simulink model "ThreePhaseInverter"  (R2020a)
settings: Solver=VariableStepAuto  StartTime=0.0  StopTime=0.1  RelTol=1e-3
libraries: powerlib x15, powerlib_meascontrol x6, simulink x4
settings Model: Creator=anif4  LastModifiedBy=anif4

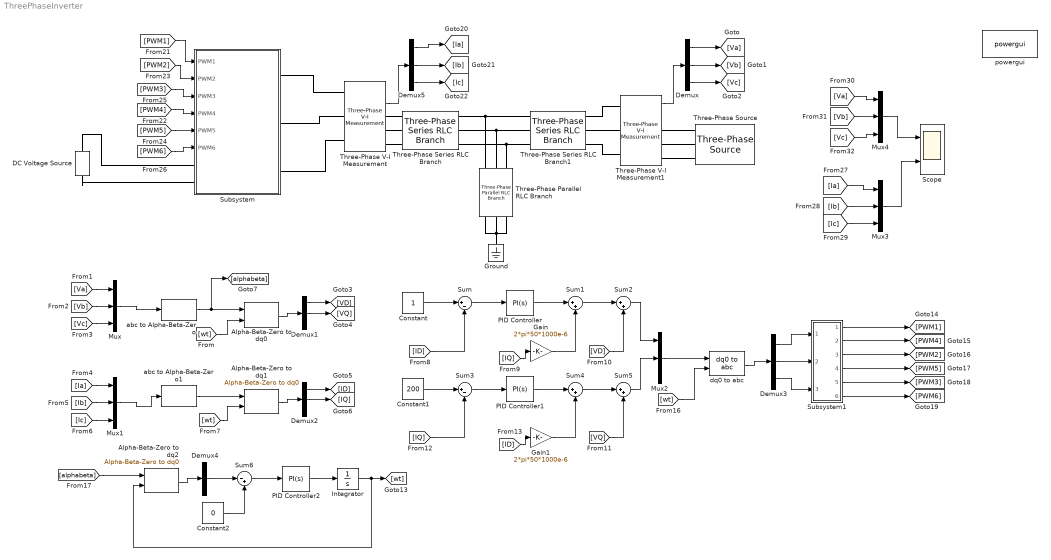
== system ThreePhaseInverter ==
  Alpha-Beta-Zero to dq0 : powerlib_meascontrol/Transformations/Alpha-Beta-Zero to dq0  Alignment=90 degrees behind phase A axis
  Alpha-Beta-Zero to dq1 : powerlib_meascontrol/Transformations/Alpha-Beta-Zero to dq0  Alignment=90 degrees behind phase A axis
  Alpha-Beta-Zero to dq2 : powerlib_meascontrol/Transformations/Alpha-Beta-Zero to dq0  Alignment=90 degrees behind phase A axis
  Constant : Constant
  Constant1 : Constant  Value=200
  Constant2 : Constant  Value=0
  DC Voltage Source : powerlib/Electrical Sources/DC Voltage Source  Amplitude=800  Measurements=None
  Demux{,1..5} (6 alike) : Demux  Outputs=3
  Gain : Gain  Gain=2*pi*50*1000e-6
  Gain1 : Gain  Gain=2*pi*50*1000e-6
  Ground : powerlib/Elements/Ground  LConnTagsString=a
  Integrator : Integrator
  Mux{,1..4} (5 alike) : Mux  Inputs=3
  PID Controller : simulink/Continuous/PID Controller  Controller=PI  Form=Parallel  TimeDomain=Continuous-time  UseExternalTs=off  SampleTime=-1  IntegratorMethod=Forward Euler  FilterMethod=Forward Euler  ControllerParametersSource=internal  P=5  I=5000  D=0  UseFilter=on  N=100  TunerSelectOption=Transfer Function Based (PID Tuner App)  InitialConditionSource=internal  InitialConditionForIntegrator=0  InitialConditionForFilter=0  DifferentiatorICPrevScaledInput=0  ExternalReset=none  TrackingMode=off  Kt=1  LimitOutput=off  UpperSaturationLimit=inf  LowerSaturationLimit=-inf  LinearizeAsGain=on  AntiWindupMode=none  Kb=1  POutMin=[]  POutMax=[]  IOutMin=[]  IOutMax=[]  DOutMin=[]  DOutMax=[]  NOutMin=[]  NOutMax=[]  SumOutMin=[]  SumOutMax=[]  SaturationOutMin=[]  SaturationOutMax=[]  PParamMin=[]  PParamMax=[]  IParamMin=[]  IParamMax=[]  DParamMin=[]  DParamMax=[]  NParamMin=[]  NParamMax=[]  KbParamMin=[]  KbParamMax=[]  KtParamMin=[]  KtParamMax=[]  KbOutMin=[]  KbOutMax=[]  KtOutMin=[]  KtOutMax=[]  IntegratorOutMin=[]  IntegratorOutMax=[]  FilterOutMin=[]  FilterOutMax=[]  SumI1OutMin=[]  SumI1OutMax=[]  SumI2OutMin=[]  SumI2OutMax=[]  SumI3OutMin=[]  SumI3OutMax=[]  SumI4OutMin=[]  SumI4OutMax=[]  SumDOutMin=[]  SumDOutMax=[]  DifferentiatorOutMin=[]  DifferentiatorOutMax=[]  FilterDiffOutCoefMin=[]  FilterDiffOutCoefMax=[]  ReciprocalOutMin=[]  ReciprocalOutMax=[]  SumDenOutMin=[]  SumDenOutMax=[]  SumNumOutMin=[]  SumNumOutMax=[]  DivideOutMin=[]  DivideOutMax=[]  UdiffTsProdOutMin=[]  UdiffTsProdOutMax=[]  NTsProdOutMin=[]  NTsProdOutMax=[]  UintegralTsProdOutMin=[]  UintegralTsProdOutMax=[]  UngainTsProdOutMin=[]  UngainTsProdOutMax=[]  IntegratorContinuousStateAttributes=''  IntegratorStateMustResolveToSignalObject=off  IntegratorRTWStateStorageClass=Auto  FilterContinuousStateAttributes=''  FilterStateMustResolveToSignalObject=off  FilterRTWStateStorageClass=Auto  ParallelPVariant=InternalParameters  IdealPVariant=Disabled  IVariant=InternalParameters  DVariant=Disabled  IntegratorVariant=Continuous  SatVariant=Disabled  AWVariant=Passthrough  PCopyVariant=Disabled  TRVariant=Disabled  FdbkBlocksVariant=Forward  IdealPFdbkVariant=Disabled  SatFdbkVariant=Disabled  DerivativeFilterVariant=Disabled  NVariant=Disabled  NCopyVariant=Disabled_SignalSpec  FilterICVariant=Disabled  IntegratorICVariant=InternalICs  ExternalResetVariant=Disabled  TRSumVariant=Passthrough  SumFdbkVariant=Disabled  SumVariant=Sum_PI  TsampFilterVariant=InternalTs  TsampNgainVariant=Passthrough  TsampIntegralVariant=Passthrough
  PID Controller1 : simulink/Continuous/PID Controller  Controller=PI  Form=Parallel  TimeDomain=Continuous-time  UseExternalTs=off  SampleTime=-1  IntegratorMethod=Forward Euler  FilterMethod=Forward Euler  ControllerParametersSource=internal  P=5  I=5000  D=0  UseFilter=on  N=100  TunerSelectOption=Transfer Function Based (PID Tuner App)  InitialConditionSource=internal  InitialConditionForIntegrator=0  InitialConditionForFilter=0  DifferentiatorICPrevScaledInput=0  ExternalReset=none  TrackingMode=off  Kt=1  LimitOutput=off  UpperSaturationLimit=inf  LowerSaturationLimit=-inf  LinearizeAsGain=on  AntiWindupMode=none  Kb=1  POutMin=[]  POutMax=[]  IOutMin=[]  IOutMax=[]  DOutMin=[]  DOutMax=[]  NOutMin=[]  NOutMax=[]  SumOutMin=[]  SumOutMax=[]  SaturationOutMin=[]  SaturationOutMax=[]  PParamMin=[]  PParamMax=[]  IParamMin=[]  IParamMax=[]  DParamMin=[]  DParamMax=[]  NParamMin=[]  NParamMax=[]  KbParamMin=[]  KbParamMax=[]  KtParamMin=[]  KtParamMax=[]  KbOutMin=[]  KbOutMax=[]  KtOutMin=[]  KtOutMax=[]  IntegratorOutMin=[]  IntegratorOutMax=[]  FilterOutMin=[]  FilterOutMax=[]  SumI1OutMin=[]  SumI1OutMax=[]  SumI2OutMin=[]  SumI2OutMax=[]  SumI3OutMin=[]  SumI3OutMax=[]  SumI4OutMin=[]  SumI4OutMax=[]  SumDOutMin=[]  SumDOutMax=[]  DifferentiatorOutMin=[]  DifferentiatorOutMax=[]  FilterDiffOutCoefMin=[]  FilterDiffOutCoefMax=[]  ReciprocalOutMin=[]  ReciprocalOutMax=[]  SumDenOutMin=[]  SumDenOutMax=[]  SumNumOutMin=[]  SumNumOutMax=[]  DivideOutMin=[]  DivideOutMax=[]  UdiffTsProdOutMin=[]  UdiffTsProdOutMax=[]  NTsProdOutMin=[]  NTsProdOutMax=[]  UintegralTsProdOutMin=[]  UintegralTsProdOutMax=[]  UngainTsProdOutMin=[]  UngainTsProdOutMax=[]  IntegratorContinuousStateAttributes=''  IntegratorStateMustResolveToSignalObject=off  IntegratorRTWStateStorageClass=Auto  FilterContinuousStateAttributes=''  FilterStateMustResolveToSignalObject=off  FilterRTWStateStorageClass=Auto  ParallelPVariant=InternalParameters  IdealPVariant=Disabled  IVariant=InternalParameters  DVariant=Disabled  IntegratorVariant=Continuous  SatVariant=Disabled  AWVariant=Passthrough  PCopyVariant=Disabled  TRVariant=Disabled  FdbkBlocksVariant=Forward  IdealPFdbkVariant=Disabled  SatFdbkVariant=Disabled  DerivativeFilterVariant=Disabled  NVariant=Disabled  NCopyVariant=Disabled_SignalSpec  FilterICVariant=Disabled  IntegratorICVariant=InternalICs  ExternalResetVariant=Disabled  TRSumVariant=Passthrough  SumFdbkVariant=Disabled  SumVariant=Sum_PI  TsampFilterVariant=InternalTs  TsampNgainVariant=Passthrough  TsampIntegralVariant=Passthrough
  PID Controller2 : simulink/Continuous/PID Controller  Controller=PI  Form=Parallel  TimeDomain=Continuous-time  UseExternalTs=off  SampleTime=-1  IntegratorMethod=Forward Euler  FilterMethod=Forward Euler  ControllerParametersSource=internal  P=50  I=50000  D=0  UseFilter=on  N=100  TunerSelectOption=Transfer Function Based (PID Tuner App)  InitialConditionSource=internal  InitialConditionForIntegrator=0  InitialConditionForFilter=0  DifferentiatorICPrevScaledInput=0  ExternalReset=none  TrackingMode=off  Kt=1  LimitOutput=off  UpperSaturationLimit=inf  LowerSaturationLimit=-inf  LinearizeAsGain=on  AntiWindupMode=none  Kb=1  POutMin=[]  POutMax=[]  IOutMin=[]  IOutMax=[]  DOutMin=[]  DOutMax=[]  NOutMin=[]  NOutMax=[]  SumOutMin=[]  SumOutMax=[]  SaturationOutMin=[]  SaturationOutMax=[]  PParamMin=[]  PParamMax=[]  IParamMin=[]  IParamMax=[]  DParamMin=[]  DParamMax=[]  NParamMin=[]  NParamMax=[]  KbParamMin=[]  KbParamMax=[]  KtParamMin=[]  KtParamMax=[]  KbOutMin=[]  KbOutMax=[]  KtOutMin=[]  KtOutMax=[]  IntegratorOutMin=[]  IntegratorOutMax=[]  FilterOutMin=[]  FilterOutMax=[]  SumI1OutMin=[]  SumI1OutMax=[]  SumI2OutMin=[]  SumI2OutMax=[]  SumI3OutMin=[]  SumI3OutMax=[]  SumI4OutMin=[]  SumI4OutMax=[]  SumDOutMin=[]  SumDOutMax=[]  DifferentiatorOutMin=[]  DifferentiatorOutMax=[]  FilterDiffOutCoefMin=[]  FilterDiffOutCoefMax=[]  ReciprocalOutMin=[]  ReciprocalOutMax=[]  SumDenOutMin=[]  SumDenOutMax=[]  SumNumOutMin=[]  SumNumOutMax=[]  DivideOutMin=[]  DivideOutMax=[]  UdiffTsProdOutMin=[]  UdiffTsProdOutMax=[]  NTsProdOutMin=[]  NTsProdOutMax=[]  UintegralTsProdOutMin=[]  UintegralTsProdOutMax=[]  UngainTsProdOutMin=[]  UngainTsProdOutMax=[]  IntegratorContinuousStateAttributes=''  IntegratorStateMustResolveToSignalObject=off  IntegratorRTWStateStorageClass=Auto  FilterContinuousStateAttributes=''  FilterStateMustResolveToSignalObject=off  FilterRTWStateStorageClass=Auto  ParallelPVariant=InternalParameters  IdealPVariant=Disabled  IVariant=InternalParameters  DVariant=Disabled  IntegratorVariant=Continuous  SatVariant=Disabled  AWVariant=Passthrough  PCopyVariant=Disabled  TRVariant=Disabled  FdbkBlocksVariant=Forward  IdealPFdbkVariant=Disabled  SatFdbkVariant=Disabled  DerivativeFilterVariant=Disabled  NVariant=Disabled  NCopyVariant=Disabled_SignalSpec  FilterICVariant=Disabled  IntegratorICVariant=InternalICs  ExternalResetVariant=Disabled  TRSumVariant=Passthrough  SumFdbkVariant=Disabled  SumVariant=Sum_PI  TsampFilterVariant=InternalTs  TsampNgainVariant=Passthrough  TsampIntegralVariant=Passthrough
  Scope : Scope  NumInputPorts=2
  Subsystem : Subsystem
  Subsystem1 : Subsystem
  Sum : Sum  Inputs=|+-
  Sum{1..2,4..5} (4 alike) : Sum  Inputs=|++
  Sum3 : Sum  Inputs=|+-
  Sum6 : Sum  Inputs=|-+
  Three-Phase Parallel RLC Branch : powerlib/Elements/Three-Phase Parallel RLC Branch  LConnTagsString=A|B|C  RConnTagsString=A|B|C  BranchType=C  Resistance=1  Inductance=1e-3  Capacitance=10e-6  Measurements=None
      settings: SourceProductBaseCode=PS
  Three-Phase Series RLC Branch : powerlib/Elements/Three-Phase Series RLC Branch  LConnTagsString=A|B|C  RConnTagsString=A|B|C  BranchType=L  Resistance=1  Inductance=5.1e-3  Capacitance=1e-6  Measurements=None
  Three-Phase Series RLC Branch1 : powerlib/Elements/Three-Phase Series RLC Branch  LConnTagsString=A|B|C  RConnTagsString=A|B|C  BranchType=L  Resistance=1  Inductance=5.1e-3  Capacitance=1e-6  Measurements=None
  Three-Phase V-I Measurement : powerlib/Measurements/Three-Phase V-I Measurement  VoltageMeasurement=phase-to-ground  SetLabelV=off  LabelV=Vabc  Vpu=off  VpuLL=off  CurrentMeasurement=yes  SetLabelI=off  LabelI=Iabc  Ipu=off  Pbase=100e6  Vbase=500e3  OutputType=Complex  PhasorSimulation=off  PSBequivalent=0
  Three-Phase V-I Measurement1 : powerlib/Measurements/Three-Phase V-I Measurement  VoltageMeasurement=phase-to-ground  SetLabelV=off  LabelV=Vabc  Vpu=off  VpuLL=off  CurrentMeasurement=yes  SetLabelI=off  LabelI=Iabc  Ipu=off  Pbase=100e6  Vbase=500e3  OutputType=Complex  PhasorSimulation=off  PSBequivalent=0
  Three-Phase Source : powerlib/Electrical Sources/Three-Phase Source  InternalConnection=Yg  VoltagePhases=off  Voltage=415  PhaseAngle=0  Voltage_phases=[25e3 25e3 25e3]/sqrt(3)  PhaseAngles_phases=[0 -120 +120]  Frequency=50  NonIdealSource=on  SpecifyImpedance=off  Resistance=0.001e-3  Inductance=16.58e-9  ShortCircuitLevel=100e6  BaseVoltage=415  XRratio=7  BusType=swing  Pref=10e3  Qref=0  Prefabc=[10e3, 10e3, 10e3]  Qrefabc=[0, 0, 0]  Qmin=-inf  Qmax=inf
  abc to Alpha-Beta-Zero : powerlib_meascontrol/Transformations/abc to Alpha-Beta-Zero
  abc to Alpha-Beta-Zero1 : powerlib_meascontrol/Transformations/abc to Alpha-Beta-Zero
  dq0 to abc : powerlib_meascontrol/Transformations/dq0 to abc  Alignment=90 degrees behind phase A axis
  powergui : powerlib/powergui  Priority=1  SimulationMode=Discrete  SampleTime=1e-6  frequency=60  Iterations=50  frequencyindice=50  Pbase=100e6  ErrMax=1e-4  UnitsV=kV  UnitsW=MW  buscounter=0  FunctionMessages=off  echomessages=off  EnableUseOfTLC=off  CurrentSourceSwitches=off  DisableSnubberDevices=off  DisableRonSwitches=off  DisableVfSwitches=off  DisplayEquations=off  AutomaticDiscreteSolvers=off  SolverType=Tustin/Backward Euler (TBE)  Interpol=off  ExternalGateDelay=off  methode=off  Ts=100  x0status=blocks  SPID=on  SwTol=0  HookPort=off  NonlinearTolerance=1e-4  nMaxIteration=100  ContinueOnMaxIteration=off  RestoreLinks=warning  ResistiveCurrentMeasurement=off  Frange=[0:2:500]  Ylog=off  Xlog=on  ShowGrid=off  save=off  variable=ZData  structure=0  ZoomFFT=off  StartTime=0.0  cycles=1  DisplayStyle=1  fundamental=60  FreqAxis=off  MaxFrequency=1000  frequencyindicesteady=1  RmsSteady=1  display=off
  wires:
  Three-Phase V-I Measurement1/1 -> Demux/1
  Demux/1 -> [Va]
  Demux/3 -> [Vc]
  Demux/2 -> [Vb]
  abc to Alpha-Beta-Zero/1 -> [alphabeta], Alpha-Beta-Zero to dq0/1
  Mux/1 -> abc to Alpha-Beta-Zero/1
  Alpha-Beta-Zero to dq0/1 -> Demux1/1
  Demux1/1 -> [VD]
  Demux1/2 -> [VQ]
  [wt] -> Alpha-Beta-Zero to dq0/2
  [Va] -> Mux/1
  [Vb] -> Mux/2
  [Vc] -> Mux/3
  [Ic] -> Mux1/3
  [Ib] -> Mux1/2
  [Ia] -> Mux1/1
  Mux1/1 -> abc to Alpha-Beta-Zero1/1
  [wt] -> Alpha-Beta-Zero to dq1/2
  Demux2/2 -> [IQ]
  Demux2/1 -> [ID]
  Alpha-Beta-Zero to dq1/1 -> Demux2/1
  abc to Alpha-Beta-Zero1/1 -> Alpha-Beta-Zero to dq1/1
  Constant/1 -> Sum/1
  [ID] -> Sum/2
  Sum/1 -> PID Controller/1
  PID Controller/1 -> Sum1/1
  Gain/1 -> Sum1/2
  [IQ] -> Gain/1
  Sum1/1 -> Sum2/1
  [VD] -> Sum2/2
  [VQ] -> Sum5/2
  Sum4/1 -> Sum5/1
  [ID] -> Gain1/1
  Gain1/1 -> Sum4/2
  PID Controller1/1 -> Sum4/1
  Sum3/1 -> PID Controller1/1
  [IQ] -> Sum3/2
  Constant1/1 -> Sum3/1
  dq0 to abc/1 -> Demux3/1
  Mux2/1 -> dq0 to abc/1
  Sum2/1 -> Mux2/1
  Sum5/1 -> Mux2/2
  [wt] -> dq0 to abc/2
  [alphabeta] -> Alpha-Beta-Zero to dq2/1
  Alpha-Beta-Zero to dq2/1 -> Demux4/1
  Demux4/2 -> Sum6/1
  Integrator/1 -> Alpha-Beta-Zero to dq2/2, [wt]
  Constant2/1 -> Sum6/2
  Sum6/1 -> PID Controller2/1
  PID Controller2/1 -> Integrator/1
  Subsystem1/1(Out1) -> [PWM1]
  Subsystem1/2(Out2) -> [PWM4]
  Subsystem1/3(Out3) -> [PWM2]
  Subsystem1/4(Out4) -> [PWM5]
  Subsystem1/5(Out5) -> [PWM3]
  Subsystem1/6(Out6) -> [PWM6]
  [PWM1] -> Subsystem/1(PWM1)
  [PWM2] -> Subsystem/2(PWM2)
  [PWM4] -> Subsystem/4(PWM4)
  [PWM3] -> Subsystem/3(PWM3)
  [PWM5] -> Subsystem/5(PWM5)
  [PWM6] -> Subsystem/6(PWM6)
  Demux5/2 -> [Ib]
  Demux5/1 -> [Ia]
  Three-Phase V-I Measurement/2 -> Demux5/1
  [Ib] -> Mux3/2
  [Ic] -> Mux3/3
  [Ia] -> Mux3/1
  [Vb] -> Mux4/2
  [Vc] -> Mux4/3
  [Va] -> Mux4/1
  Mux4/1 -> Scope/1
  Mux3/1 -> Scope/2
  Demux5/3 -> [Ic]
  Demux3/1 -> Subsystem1/1(In1)
  Demux3/2 -> Subsystem1/2(In2)
  Demux3/3 -> Subsystem1/3(In3)
  connections:
  DC Voltage Source/RConn1 -- Subsystem/LConn1
  DC Voltage Source/LConn1 -- Subsystem/LConn2
  Subsystem/RConn1 -- Three-Phase V-I Measurement/LConn1
  Subsystem/RConn2 -- Three-Phase V-I Measurement/LConn2
  Subsystem/RConn3 -- Three-Phase V-I Measurement/LConn3
  Three-Phase Series RLC Branch/LConn3 -- Three-Phase V-I Measurement/RConn3
  Three-Phase V-I Measurement/RConn2 -- Three-Phase Series RLC Branch/LConn2
  Three-Phase V-I Measurement/RConn1 -- Three-Phase Series RLC Branch/LConn1
  Three-Phase Series RLC Branch/RConn3 -- Three-Phase Series RLC Branch1/LConn3 -- Three-Phase Parallel RLC Branch/LConn3
  Three-Phase Series RLC Branch1/LConn2 -- Three-Phase Parallel RLC Branch/LConn2 -- Three-Phase Series RLC Branch/RConn2
  Three-Phase Series RLC Branch/RConn1 -- Three-Phase Series RLC Branch1/LConn1 -- Three-Phase Parallel RLC Branch/LConn1
  Three-Phase Parallel RLC Branch/RConn3 -- Three-Phase Parallel RLC Branch/RConn2 -- Ground/LConn1 -- Three-Phase Parallel RLC Branch/RConn1
  Three-Phase V-I Measurement1/LConn2 -- Three-Phase Series RLC Branch1/RConn2
  Three-Phase Series RLC Branch1/RConn1 -- Three-Phase V-I Measurement1/LConn1
  Three-Phase Series RLC Branch1/RConn3 -- Three-Phase V-I Measurement1/LConn3
  Three-Phase Source/RConn2 -- Three-Phase V-I Measurement1/RConn2
  Three-Phase Source/RConn1 -- Three-Phase V-I Measurement1/RConn3
  Three-Phase Source/RConn3 -- Three-Phase V-I Measurement1/RConn1

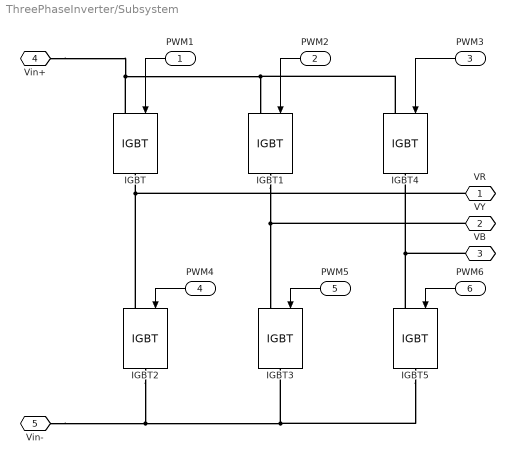
== system ThreePhaseInverter/Subsystem ==
  PWM1 : Inport
  PWM2 : Inport  Port=2
  PWM3 : Inport  Port=3
  PWM4 : Inport  Port=4
  PWM5 : Inport  Port=5
  PWM6 : Inport  Port=6
  IGBT{,1..5} (6 alike) : powerlib/Power Electronics/IGBT  Ron=0.001  Lon=0  Vf=1  Tf=1e-6  Tt=2e-6  IC=0  Rs=1e5  Cs=inf  Measurements=off
  VR : PMIOPort  Side=Right
  VY : PMIOPort  Port=2  Side=Right
  VB : PMIOPort  Port=3  Side=Right
  Vin+ : PMIOPort  Port=4  Side=Left
  Vin- : PMIOPort  Port=5  Side=Left
  wires:
  PWM6/1 -> IGBT5/1
  PWM2/1 -> IGBT1/1
  PWM3/1 -> IGBT4/1
  PWM5/1 -> IGBT3/1
  PWM4/1 -> IGBT2/1
  PWM1/1 -> IGBT/1
  connections:
  IGBT/LConn1 -- Vin+/RConn1 -- IGBT4/LConn1 -- IGBT1/LConn1
  IGBT2/RConn1 -- Vin-/RConn1 -- IGBT5/RConn1 -- IGBT3/RConn1
  IGBT1/RConn1 -- VY/RConn1 -- IGBT3/LConn1
  IGBT5/LConn1 -- VB/RConn1 -- IGBT4/RConn1
  IGBT2/LConn1 -- VR/RConn1 -- IGBT/RConn1

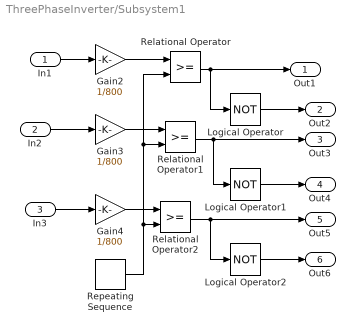
== system ThreePhaseInverter/Subsystem1 ==
  In1 : Inport
  In2 : Inport  Port=2
  In3 : Inport  Port=3
  Gain2 : Gain  Gain=1/800
  Gain3 : Gain  Gain=1/800
  Gain4 : Gain  Gain=1/800
  Logical Operator : Logic  Operator=NOT  AllPortsSameDT=off  OutDataTypeStr=boolean
  Logical Operator1 : Logic  Operator=NOT  AllPortsSameDT=off  OutDataTypeStr=boolean
  Logical Operator2 : Logic  Operator=NOT  AllPortsSameDT=off  OutDataTypeStr=boolean
  Relational Operator : RelationalOperator  OutDataTypeStr=boolean  RndMeth=Simplest
  Relational Operator1 : RelationalOperator  OutDataTypeStr=boolean  RndMeth=Simplest
  Relational Operator2 : RelationalOperator  OutDataTypeStr=boolean  RndMeth=Simplest
  Repeating Sequence : simulink/Sources/Repeating Sequence  rep_seq_t=[0 0.00005 0.0001]  rep_seq_y=[-1 1 -1]
  Out1 : Outport
  Out2 : Outport  Port=2
  Out3 : Outport  Port=3
  Out4 : Outport  Port=4
  Out5 : Outport  Port=5
  Out6 : Outport  Port=6
  wires:
  Gain2/1 -> Relational Operator/1
  Repeating Sequence/1 -> Relational Operator/2, Relational Operator1/2, Relational Operator2/2
  Relational Operator2/1 -> Out5/1, Logical Operator2/1
  Logical Operator1/1 -> Out4/1
  In1/1 -> Gain2/1
  Relational Operator/1 -> Out1/1, Logical Operator/1
  Gain3/1 -> Relational Operator1/1
  Relational Operator1/1 -> Out3/1, Logical Operator1/1
  Gain4/1 -> Relational Operator2/1
  In2/1 -> Gain3/1
  In3/1 -> Gain4/1
  Logical Operator2/1 -> Out6/1
  Logical Operator/1 -> Out2/1
